simulink model "motor_pos"  (R2020b)
settings: Solver=ode15s  StartTime=0.0  StopTime=0.2  RelTol=1e-3
undefined symbols (not defined in the file): b, J, K, L, R
settings Model: Creator=priyaD  LastModifiedBy=priyaD

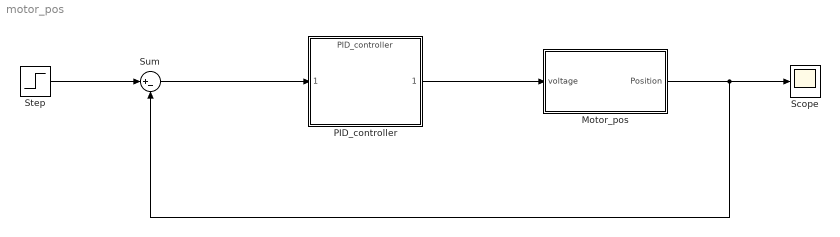
== system motor_pos ==
  Motor_pos : Subsystem  TreatAsAtomicUnit=on
  PID_controller : ModelReference  ModelNameDialog=PID_controller  ModelReferenceVersion=1.15
  Scope : Scope
  Step : Step  Time=0.001  SampleTime=0
  Sum : Sum  Inputs=|+-
  wires:
  Step/1 -> Sum/1
  Sum/1 -> PID_controller/1
  PID_controller/1 -> Motor_pos/1(voltage)
  Motor_pos/1(Position) -> Sum/2, Scope/1

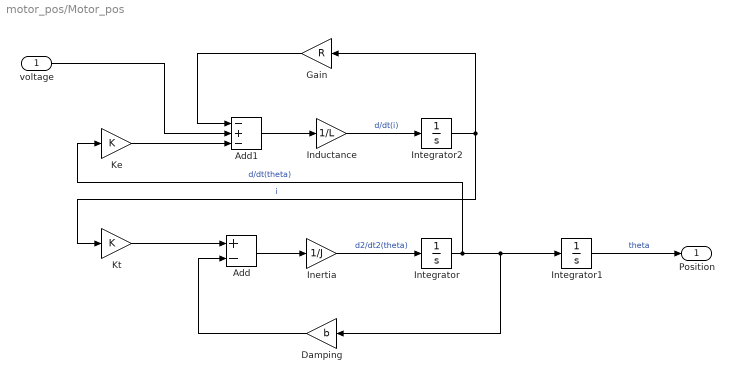
== system motor_pos/Motor_pos ==
  voltage : Inport
  Add : Sum  Inputs=+-
  Add1 : Sum  Inputs=-+-
  Damping : Gain  Gain=b
  Gain : Gain  Gain=R
  Inductance : Gain  Gain=1/L
  Inertia : Gain  Gain=1/J
  Integrator : Integrator
  Integrator1 : Integrator
  Integrator2 : Integrator
  Ke : Gain  Gain=K
  Kt : Gain  Gain=K
  Position : Outport
  wires:
  Damping/1 -> Add/2
  Integrator/1 -> Ke/1, Damping/1, Integrator1/1  "d/dt(theta)"
  Gain/1 -> Add1/1
  Add/1 -> Inertia/1
  Kt/1 -> Add/1
  Inertia/1 -> Integrator/1  "d2/dt2(theta)"
  Add1/1 -> Inductance/1
  voltage/1 -> Add1/2
  Integrator2/1 -> Gain/1, Kt/1  "i"
  Ke/1 -> Add1/3
  Inductance/1 -> Integrator2/1  "d/dt(i)"
  Integrator1/1 -> Position/1  "theta"
